simulink model "DisplayVideo"  (R2020a)
settings: Solver=FixedStepDiscrete  StartTime=0.0  StopTime=30  FixedStep=1/5  RelTol=1e-3
undefined symbols (not defined in the file or in its folder): gray
libraries: simulink_extras x1
settings Model: EnablePacing=on  Creator=kelvinxie  LastModifiedBy=kelvinxie

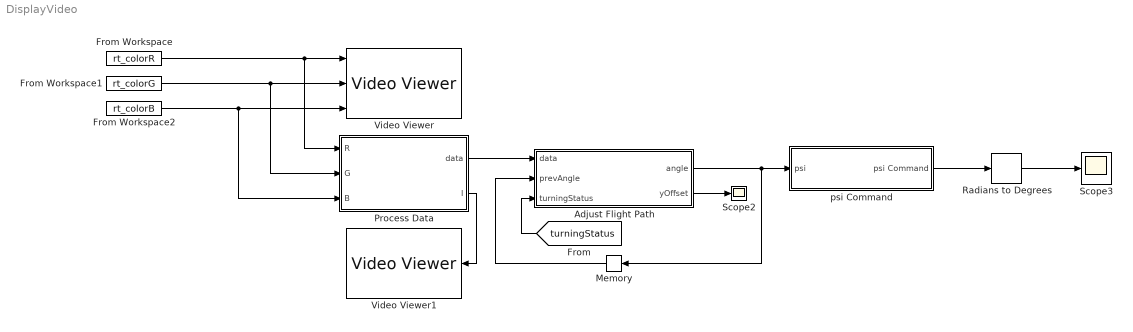
== system DisplayVideo ==
  Adjust Flight Path : MATLAB Function  TreatAsAtomicUnit=on
  From Workspace : FromWorkspace  VariableName=rt_colorR
  From Workspace1 : FromWorkspace  VariableName=rt_colorG
  From Workspace2 : FromWorkspace  VariableName=rt_colorB
  Memory : Memory  InitialCondition=-pi/2
  Process Data : MATLAB Function  TreatAsAtomicUnit=on
  Radians to Degrees : simulink_extras/Transformations/Radians to Degrees
  Scope2 : Scope
  Scope3 : Scope
  Video Viewer : VideoViewer  imagePorts=separate color signals  colormapValue=gray(256)  FigPos=[1 1438 1274 1363]
  Video Viewer1 : VideoViewer  colormapValue=gray(256)  FigPos=[1287 1438 1274 1363]
  psi Command : Subsystem
  wires:
  From Workspace1/1 -> Process Data/2(G), Video Viewer/2
  From Workspace2/1 -> Process Data/3(B), Video Viewer/3
  From Workspace/1 -> Process Data/1(R), Video Viewer/1
  Process Data/1(data) -> Adjust Flight Path/1(data)
  Process Data/2(I) -> Video Viewer1/1
  Memory/1 -> Adjust Flight Path/2(prevAngle)
  Adjust Flight Path/2(yOffset) -> Scope2/1
  psi Command/1(psi Command) -> Radians to Degrees/1
  Adjust Flight Path/1(angle) -> Memory/1, psi Command/1(psi)
  Radians to Degrees/1 -> Scope3/1
  [turningStatus] -> Adjust Flight Path/3(turningStatus)

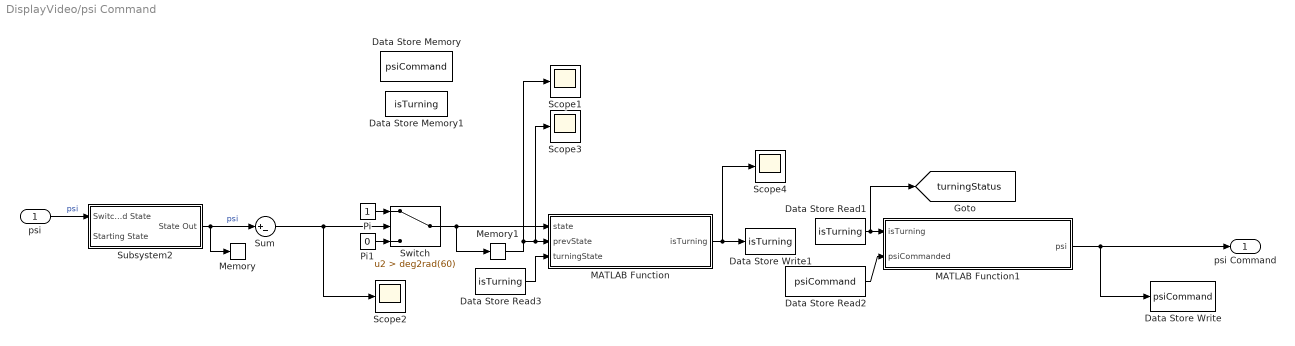
== system DisplayVideo/psi Command ==
  psi : Inport
  Data Store Memory : DataStoreMemory  DataStoreName=psiCommand  ReadBeforeWriteMsg=warning  WriteAfterWriteMsg=warning  WriteAfterReadMsg=warning  ShowAdditionalParam=off
  Data Store Memory1 : DataStoreMemory  DataStoreName=isTurning  ReadBeforeWriteMsg=warning  WriteAfterWriteMsg=warning  WriteAfterReadMsg=warning  ShowAdditionalParam=off
  Data Store Read1 : DataStoreRead  DataStoreName=isTurning
  Data Store Read2 : DataStoreRead  DataStoreName=psiCommand
  Data Store Read3 : DataStoreRead  DataStoreName=isTurning
  Data Store Write : DataStoreWrite  DataStoreName=psiCommand
  Data Store Write1 : DataStoreWrite  DataStoreName=isTurning
  MATLAB Function : MATLAB Function  TreatAsAtomicUnit=on
  MATLAB Function1 : MATLAB Function  TreatAsAtomicUnit=on
  Memory : Memory  InheritSampleTime=on
  Memory1 : Memory  InheritSampleTime=on
  Pi : Constant  OutDataTypeStr=Inherit: Inherit via back propagation
  Pi1 : Constant  Value=0  OutDataTypeStr=Inherit: Inherit via back propagation
  Scope{1..4} (4 alike) : Scope
  Subsystem2 : Subsystem
  Sum : Sum  Inputs=|+-
  Switch : Switch  Criteria=u2 > Threshold  Threshold=deg2rad(60)
  psi Command : Outport
  tag scope: turningStatus=global
  wires:
  psi/1 -> Subsystem2/1(Switched State)  "psi"
  Subsystem2/1(State Out) -> Sum/1, Memory/1  "psi"
  Pi/1 -> Switch/1
  Pi1/1 -> Switch/3
  MATLAB Function1/1(psi) -> psi Command/1, Data Store Write/1
  Switch/1 -> Memory1/1, MATLAB Function/1(state)
  Memory1/1 -> Scope1/1, Scope3/1, MATLAB Function/2(prevState)
  MATLAB Function/1(isTurning) -> Scope4/1, Data Store Write1/1
  Data Store Read1/1 -> [turningStatus], MATLAB Function1/1(isTurning)
  Data Store Read2/1 -> MATLAB Function1/2(psiCommanded)
  Sum/1 -> Switch/2, Scope2/1
  Data Store Read3/1 -> MATLAB Function/3(turningState)

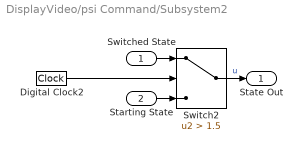
== system DisplayVideo/psi Command/Subsystem2 ==
  Switched State : Inport
  Starting State : Inport  Port=2
  Digital Clock2 : DigitalClock  SampleTime=1/5
  Switch2 : Switch  Criteria=u2 > Threshold  Threshold=1.5
  State Out : Outport
  wires:
  Switched State/1 -> Switch2/1
  Starting State/1 -> Switch2/3
  Switch2/1 -> State Out/1  "u"
  Digital Clock2/1 -> Switch2/2

== matlab function DisplayVideo/psi Command/MATLAB Function1 ==
  data: isTurning input; psi output; psiCommanded input
function psi = changePsi(isTurning, psiCommanded)
    if isTurning == 1
        psi = psiCommanded + pi/2; % adds pi/2 to the commanded psi angle
    else
        psi = psiCommanded;
    end
end

== matlab function DisplayVideo/psi Command/MATLAB Function ==
  settings: updateMethod=DISCRETE
  data: state input; isTurning output; prevState input; turningState input
function isTurning = turningState(state, prevState, turningState)
    if state == 1 && prevState == 0 
        isTurning = 1; %entering turn
    elseif state == 0 && prevState == 1 && turningState == 1/2
        isTurning = 0; %exiting turn
    elseif state == 1 && prevState == 1
        isTurning = 1/2;
    else
        isTurning = 0;
    end
end

== matlab function DisplayVideo/Process Data ==
  settings: updateMethod=DISCRETE  sampleTime=1/5
  data: R input; G input; B input; data output size=[2 2000]; I output
function [data,I] = processData(R, G, B)
picture = cat(3,R,G,B);
greyImage = rgb2gray(picture);
I = edge(greyImage, 'sobel', 0.15);
I(:, [1:10, 150:160]) = 0;
topHalf = I(1:60, :);
topHalf(:, [1:40, 120:160]) = 0;
[y x] = find(topHalf);
x = x - 80;
y = -y + 60;
data = [x'; y'];
end

== matlab function DisplayVideo/Adjust Flight Path ==
  settings: updateMethod=DISCRETE  sampleTime=1/5
  data: angle output; data input size=[2 2000]; prevAngle input; yOffset output; turningStatus input
function [angle,yOffset]  = adjustAngle(data, prevAngle, turningStatus)
    x = data(1,:);
    y = data(2,:);
    if sum(data, 'all') < 6
        angle = prevAngle;
    else
        y1 = y(1);
        y2 = y(end);
        x1 = x(1);
        x2 = x(end);
        if y1 < y2
            angle = atan2(y(end)-y(1), x(end)-x(1));
        elseif y2 < y1
            angle = atan2(y(1)-y(end), x(1)-x(end));
        else
            angle = prevAngle;
        end
        angle = angle - pi/2;
    end

    if turningStatus == 0
        yOffset = mean(x);
    else
        yOffset= 0;
    end
end
